simulink library "goose_lib"  (Simulink 8.1)
settings: Solver=ode45  StartTime=0.0  StopTime=10.0  RelTol=1e-3
undefined symbols (not defined in the file): CD, relay_iec61850
libraries: rtio_iec61850 x60
(part 2 of 2)

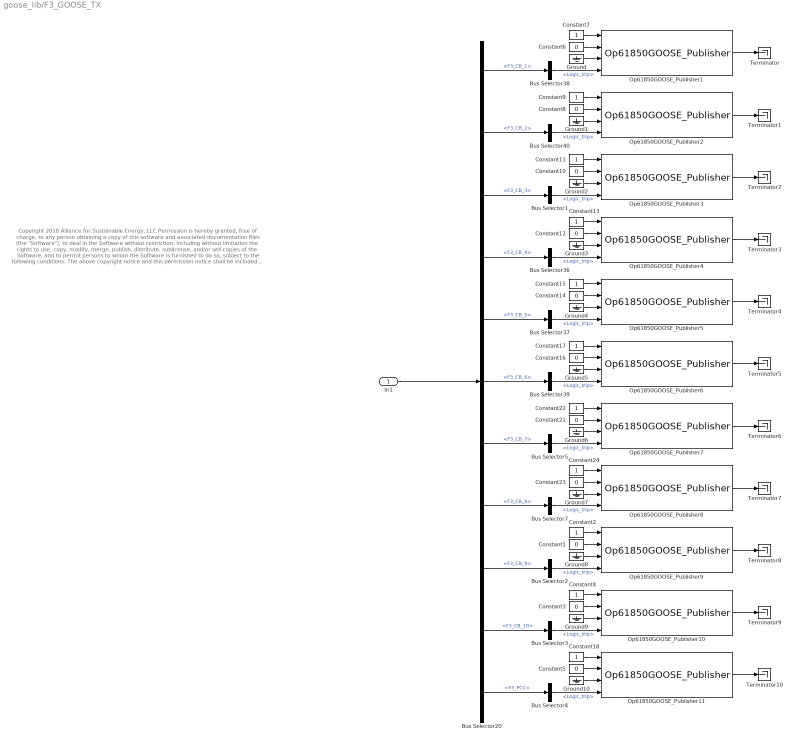
== system goose_lib/F3_GOOSE_TX ==
  note: Copyright 2018 Alliance for Sustainable Energy, LLC
      |
      | Permission is hereby granted, free of charge, to any person obtaining a copy of this software
      | and associated documentation files (the "Software"), to deal in the Software without restriction,
      | including without limitation the rights to use, copy, modify, merge, publish, distribute, sublicense,
      | and/or sell copies of the Software, and to permit persons to whom the Software is furnished to do so,
      | subject to the following conditions:
      |
      | The above copyright notice and this permission notice shall be included in all copies or substantial portions of the Software.
      |
      | THE SOFTWARE IS PROVIDED "AS IS", WITHOUT WARRANTY OF ANY KIND, EXPRESS OR IMPLIED, INCLUDING
      | BUT NOT LIMITED TO THE WARRANTIES OF MERCHANTABILITY, FITNESS FOR A PARTICULAR PURPOSE AND
      | NONINFRINGEMENT. IN NO EVENT SHALL THE AUTHORS, THE COPYRIGHT HOLDERS, THE UNITED STATES,
      | THE UNITED STATES DEPARTMENT OF ENERGY, OR ANY OF THEIR EMPLOYEES BE LIABLE FOR ANY CLAIM,
      | DAMAGES OR OTHER LIABILITY, WHETHER IN AN ACTION OF CONTRACT, TORT OR OTHERWISE, ARISING FROM,
      | OUT OF OR IN CONNECTION WITH THE SOFTWARE OR THE USE OR OTHER DEALINGS IN THE SOFTWARE.
  In1 : Inport
  Bus Selector{1..5,7,36..40} (11 alike) : BusSelector  OutputSignals=Logic_trip
  Bus Selector20 : BusSelector  OutputSignals=F3_CB_1,F3_CB_2,F3_CB_3,F3_CB_4,F3_CB_5,F3_CB_6,F3_CB_7,F3_CB_8,F3_CB_9,F3_CB_10,F3_PCC
  Constant{1,3,5..6,8,10,12,14,16,21,23} (11 alike) : Constant  Value=0
  Constant{2,4,7,9,11,13,15,17..18,22,24} (11 alike) : Constant
  Ground{,1..10} (11 alike) : Ground
  Op61850GOOSE_Publisher1 : rtio_iec61850/Op61850GOOSE_Publisher  nic_name=eth1  ied_name=CB301  select_scl=off  scl_file=CB301.icd  scl_fullpath=.\relay_iec61850  goose_name=Goose_TRIP1  goose_msgid=0x0301  mac_address=01-0C-CD-01-23-01  vlan_prio=4  vlan_id=000  mintime=25  maxtime=250  gocbref=CB301LDevice1/LLN0$GO$CB_Goose_TRIP1  dataset=CB301LDevice1/LLN0$Goose_TRIP1  goID=Goose_TRIP1  confrev=1  externalClock=off
      settings: AttributesFormatString=%<Name>\nAppId = %<goose_msgid>
  Op61850GOOSE_Publisher10 : rtio_iec61850/Op61850GOOSE_Publisher  nic_name=eth1  ied_name=CB310  select_scl=off  scl_file=CB310.icd  scl_fullpath=.\relay_iec61850  goose_name=Goose_TRIP1  goose_msgid=0x0310  mac_address=01-0C-CD-01-23-10  vlan_prio=4  vlan_id=000  mintime=25  maxtime=250  gocbref=CB310LDevice1/LLN0$GO$CB_Goose_TRIP1  dataset=CB310LDevice1/LLN0$Goose_TRIP1  goID=Goose_TRIP1  confrev=1  externalClock=off
      settings: AttributesFormatString=%<Name>\nAppId = %<goose_msgid>
  Op61850GOOSE_Publisher11 : rtio_iec61850/Op61850GOOSE_Publisher  nic_name=eth1  ied_name=CB300  select_scl=off  scl_file=CB300.icd  scl_fullpath=.\relay_iec61850  goose_name=Goose_TRIP1  goose_msgid=0x0300  mac_address=01-0C-CD-01-23-00  vlan_prio=4  vlan_id=000  mintime=25  maxtime=250  gocbref=CB300LDevice1/LLN0$GO$CB_Goose_TRIP1  dataset=CB300LDevice1/LLN0$Goose_TRIP1  goID=Goose_TRIP1  confrev=1  externalClock=off
      settings: AttributesFormatString=%<Name>\nAppId = %<goose_msgid>
  Op61850GOOSE_Publisher2 : rtio_iec61850/Op61850GOOSE_Publisher  nic_name=eth1  ied_name=CB302  select_scl=off  scl_file=CB302.icd  scl_fullpath=.\relay_iec61850  goose_name=Goose_TRIP1  goose_msgid=0x0302  mac_address=01-0C-CD-01-23-02  vlan_prio=4  vlan_id=000  mintime=25  maxtime=250  gocbref=CB302LDevice1/LLN0$GO$CB_Goose_TRIP1  dataset=CB302LDevice1/LLN0$Goose_TRIP1  goID=Goose_TRIP1  confrev=1  externalClock=off
      settings: AttributesFormatString=%<Name>\nAppId = %<goose_msgid>
  Op61850GOOSE_Publisher3 : rtio_iec61850/Op61850GOOSE_Publisher  nic_name=eth1  ied_name=CB303  select_scl=off  scl_file=CB303.icd  scl_fullpath=.\relay_iec61850  goose_name=Goose_TRIP1  goose_msgid=0x0303  mac_address=01-0C-CD-01-23-03  vlan_prio=4  vlan_id=000  mintime=25  maxtime=250  gocbref=CB303LDevice1/LLN0$GO$CB_Goose_TRIP1  dataset=CB303LDevice1/LLN0$Goose_TRIP1  goID=Goose_TRIP1  confrev=1  externalClock=off
      settings: AttributesFormatString=%<Name>\nAppId = %<goose_msgid>
  Op61850GOOSE_Publisher4 : rtio_iec61850/Op61850GOOSE_Publisher  nic_name=eth1  ied_name=CB304  select_scl=off  scl_file=CB304.icd  scl_fullpath=.\relay_iec61850  goose_name=Goose_TRIP1  goose_msgid=0x0304  mac_address=01-0C-CD-01-23-04  vlan_prio=4  vlan_id=000  mintime=25  maxtime=250  gocbref=CB304LDevice1/LLN0$GO$CB_Goose_TRIP1  dataset=CB304LDevice1/LLN0$Goose_TRIP1  goID=Goose_TRIP1  confrev=1  externalClock=off
      settings: AttributesFormatString=%<Name>\nAppId = %<goose_msgid>
  Op61850GOOSE_Publisher5 : rtio_iec61850/Op61850GOOSE_Publisher  nic_name=eth1  ied_name=CB305  select_scl=off  scl_file=CB305.icd  scl_fullpath=.\relay_iec61850  goose_name=Goose_TRIP1  goose_msgid=0x0305  mac_address=01-0C-CD-01-23-05  vlan_prio=4  vlan_id=000  mintime=25  maxtime=250  gocbref=CB305LDevice1/LLN0$GO$CB_Goose_TRIP1  dataset=CB305LDevice1/LLN0$Goose_TRIP1  goID=Goose_TRIP1  confrev=1  externalClock=off
      settings: AttributesFormatString=%<Name>\nAppId = %<goose_msgid>
  Op61850GOOSE_Publisher6 : rtio_iec61850/Op61850GOOSE_Publisher  nic_name=eth1  ied_name=CB306  select_scl=off  scl_file=CB306.icd  scl_fullpath=.\relay_iec61850  goose_name=Goose_TRIP1  goose_msgid=0x0306  mac_address=01-0C-CD-01-23-06  vlan_prio=4  vlan_id=000  mintime=25  maxtime=250  gocbref=CB306LDevice1/LLN0$GO$CB_Goose_TRIP1  dataset=CB306LDevice1/LLN0$Goose_TRIP1  goID=Goose_TRIP1  confrev=1  externalClock=off
      settings: AttributesFormatString=%<Name>\nAppId = %<goose_msgid>
  Op61850GOOSE_Publisher7 : rtio_iec61850/Op61850GOOSE_Publisher  nic_name=eth1  ied_name=CB307  select_scl=off  scl_file=CB307.icd  scl_fullpath=.\relay_iec61850  goose_name=Goose_TRIP1  goose_msgid=0x0307  mac_address=01-0C-CD-01-23-07  vlan_prio=4  vlan_id=000  mintime=25  maxtime=250  gocbref=CB307LDevice1/LLN0$GO$CB_Goose_TRIP1  dataset=CB307LDevice1/LLN0$Goose_TRIP1  goID=Goose_TRIP1  confrev=1  externalClock=off
      settings: AttributesFormatString=%<Name>\nAppId = %<goose_msgid>
  Op61850GOOSE_Publisher8 : rtio_iec61850/Op61850GOOSE_Publisher  nic_name=eth1  ied_name=CB308  select_scl=off  scl_file=CB308.icd  scl_fullpath=.\relay_iec61850  goose_name=Goose_TRIP1  goose_msgid=0x0308  mac_address=01-0C-CD-01-23-08  vlan_prio=4  vlan_id=000  mintime=25  maxtime=250  gocbref=CB308LDevice1/LLN0$GO$CB_Goose_TRIP1  dataset=CB308LDevice1/LLN0$Goose_TRIP1  goID=Goose_TRIP1  confrev=1  externalClock=off
      settings: AttributesFormatString=%<Name>\nAppId = %<goose_msgid>
  Op61850GOOSE_Publisher9 : rtio_iec61850/Op61850GOOSE_Publisher  nic_name=eth1  ied_name=CB309  select_scl=off  scl_file=CB309.icd  scl_fullpath=.\relay_iec61850  goose_name=Goose_TRIP1  goose_msgid=0x0309  mac_address=01-0C-CD-01-23-09  vlan_prio=4  vlan_id=000  mintime=25  maxtime=250  gocbref=CB309LDevice1/LLN0$GO$CB_Goose_TRIP1  dataset=CB309LDevice1/LLN0$Goose_TRIP1  goID=Goose_TRIP1  confrev=1  externalClock=off
      settings: AttributesFormatString=%<Name>\nAppId = %<goose_msgid>
  Terminator{,1..10} (11 alike) : Terminator
  wires:
  Ground5/1 -> Op61850GOOSE_Publisher6/3
  Constant17/1 -> Op61850GOOSE_Publisher6/1
  Ground3/1 -> Op61850GOOSE_Publisher4/3
  Ground1/1 -> Op61850GOOSE_Publisher2/3
  In1/1 -> Bus Selector20/1
  Constant16/1 -> Op61850GOOSE_Publisher6/2
  Bus Selector39/1 -> Op61850GOOSE_Publisher6/4  "<Logic_trip>"
  Bus Selector20/6 -> Bus Selector39/1  "<F3_CB_6>"
  Op61850GOOSE_Publisher5/1 -> Terminator4/1
  Ground4/1 -> Op61850GOOSE_Publisher5/3
  Constant12/1 -> Op61850GOOSE_Publisher4/2
  Constant13/1 -> Op61850GOOSE_Publisher4/1
  Bus Selector36/1 -> Op61850GOOSE_Publisher4/4  "<Logic_trip>"
  Bus Selector20/4 -> Bus Selector36/1  "<F3_CB_4>"
  Op61850GOOSE_Publisher3/1 -> Terminator2/1
  Constant9/1 -> Op61850GOOSE_Publisher2/1
  Constant8/1 -> Op61850GOOSE_Publisher2/2
  Bus Selector40/1 -> Op61850GOOSE_Publisher2/4  "<Logic_trip>"
  Bus Selector20/2 -> Bus Selector40/1  "<F3_CB_2>"
  Ground2/1 -> Op61850GOOSE_Publisher3/3
  Op61850GOOSE_Publisher1/1 -> Terminator/1
  Op61850GOOSE_Publisher2/1 -> Terminator1/1
  Op61850GOOSE_Publisher4/1 -> Terminator3/1
  Constant14/1 -> Op61850GOOSE_Publisher5/2
  Constant7/1 -> Op61850GOOSE_Publisher1/1
  Ground/1 -> Op61850GOOSE_Publisher1/3
  Constant11/1 -> Op61850GOOSE_Publisher3/1
  Constant10/1 -> Op61850GOOSE_Publisher3/2
  Constant15/1 -> Op61850GOOSE_Publisher5/1
  Bus Selector37/1 -> Op61850GOOSE_Publisher5/4  "<Logic_trip>"
  Bus Selector20/5 -> Bus Selector37/1  "<F3_CB_5>"
  Bus Selector38/1 -> Op61850GOOSE_Publisher1/4  "<Logic_trip>"
  Bus Selector20/1 -> Bus Selector38/1  "<F3_CB_1>"
  Bus Selector20/3 -> Bus Selector1/1  "<F3_CB_3>"
  Bus Selector1/1 -> Op61850GOOSE_Publisher3/4  "<Logic_trip>"
  Constant6/1 -> Op61850GOOSE_Publisher1/2
  Op61850GOOSE_Publisher6/1 -> Terminator5/1
  Ground9/1 -> Op61850GOOSE_Publisher10/3
  Ground7/1 -> Op61850GOOSE_Publisher8/3
  Op61850GOOSE_Publisher11/1 -> Terminator10/1
  Ground10/1 -> Op61850GOOSE_Publisher11/3
  Constant3/1 -> Op61850GOOSE_Publisher10/2
  Constant4/1 -> Op61850GOOSE_Publisher10/1
  Bus Selector3/1 -> Op61850GOOSE_Publisher10/4  "<Logic_trip>"
  Op61850GOOSE_Publisher9/1 -> Terminator8/1
  Constant24/1 -> Op61850GOOSE_Publisher8/1
  Constant23/1 -> Op61850GOOSE_Publisher8/2
  Bus Selector7/1 -> Op61850GOOSE_Publisher8/4  "<Logic_trip>"
  Ground8/1 -> Op61850GOOSE_Publisher9/3
  Op61850GOOSE_Publisher7/1 -> Terminator6/1
  Op61850GOOSE_Publisher8/1 -> Terminator7/1
  Op61850GOOSE_Publisher10/1 -> Terminator9/1
  Constant5/1 -> Op61850GOOSE_Publisher11/2
  Constant22/1 -> Op61850GOOSE_Publisher7/1
  Ground6/1 -> Op61850GOOSE_Publisher7/3
  Constant2/1 -> Op61850GOOSE_Publisher9/1
  Constant1/1 -> Op61850GOOSE_Publisher9/2
  Constant18/1 -> Op61850GOOSE_Publisher11/1
  Bus Selector4/1 -> Op61850GOOSE_Publisher11/4  "<Logic_trip>"
  Bus Selector5/1 -> Op61850GOOSE_Publisher7/4  "<Logic_trip>"
  Bus Selector2/1 -> Op61850GOOSE_Publisher9/4  "<Logic_trip>"
  Constant21/1 -> Op61850GOOSE_Publisher7/2
  Bus Selector20/10 -> Bus Selector3/1  "<F3_CB_10>"
  Bus Selector20/8 -> Bus Selector7/1  "<F3_CB_8>"
  Bus Selector20/11 -> Bus Selector4/1  "<F3_PCC>"
  Bus Selector20/7 -> Bus Selector5/1  "<F3_CB_7>"
  Bus Selector20/9 -> Bus Selector2/1  "<F3_CB_9>"

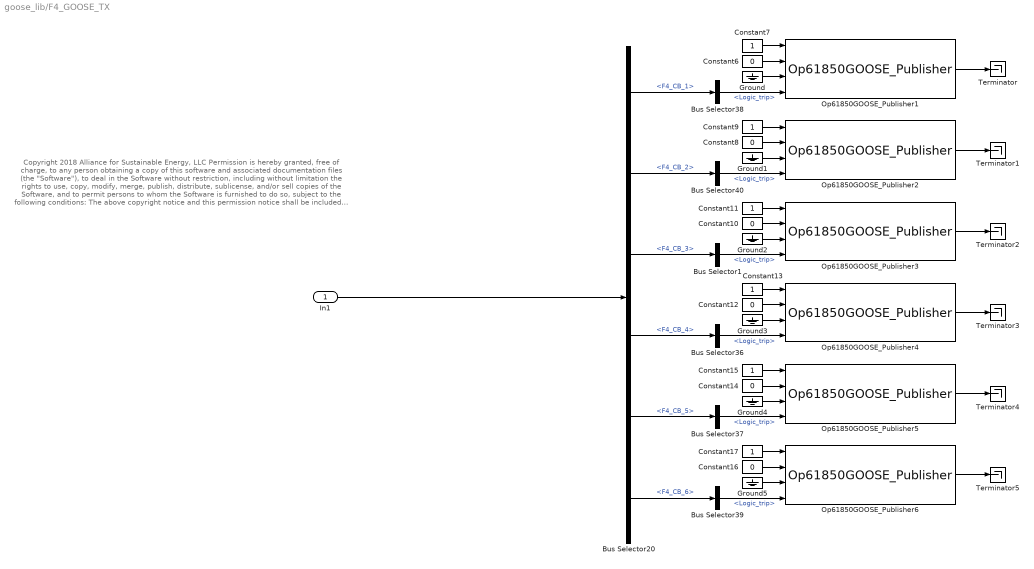
== system goose_lib/F4_GOOSE_TX ==
  note: Copyright 2018 Alliance for Sustainable Energy, LLC
      |
      | Permission is hereby granted, free of charge, to any person obtaining a copy of this software
      | and associated documentation files (the "Software"), to deal in the Software without restriction,
      | including without limitation the rights to use, copy, modify, merge, publish, distribute, sublicense,
      | and/or sell copies of the Software, and to permit persons to whom the Software is furnished to do so,
      | subject to the following conditions:
      |
      | The above copyright notice and this permission notice shall be included in all copies or substantial portions of the Software.
      |
      | THE SOFTWARE IS PROVIDED "AS IS", WITHOUT WARRANTY OF ANY KIND, EXPRESS OR IMPLIED, INCLUDING
      | BUT NOT LIMITED TO THE WARRANTIES OF MERCHANTABILITY, FITNESS FOR A PARTICULAR PURPOSE AND
      | NONINFRINGEMENT. IN NO EVENT SHALL THE AUTHORS, THE COPYRIGHT HOLDERS, THE UNITED STATES,
      | THE UNITED STATES DEPARTMENT OF ENERGY, OR ANY OF THEIR EMPLOYEES BE LIABLE FOR ANY CLAIM,
      | DAMAGES OR OTHER LIABILITY, WHETHER IN AN ACTION OF CONTRACT, TORT OR OTHERWISE, ARISING FROM,
      | OUT OF OR IN CONNECTION WITH THE SOFTWARE OR THE USE OR OTHER DEALINGS IN THE SOFTWARE.
  In1 : Inport
  Bus Selector{1,36..40} (6 alike) : BusSelector  OutputSignals=Logic_trip
  Bus Selector20 : BusSelector  OutputSignals=F4_CB_1,F4_CB_2,F4_CB_3,F4_CB_4,F4_CB_5,F4_CB_6
  Constant{6,8,10,12,14,16} (6 alike) : Constant  Value=0
  Constant{7,9,11,13,15,17} (6 alike) : Constant
  Ground{,1..5} (6 alike) : Ground
  Op61850GOOSE_Publisher1 : rtio_iec61850/Op61850GOOSE_Publisher  nic_name=eth1  ied_name=CB401  select_scl=off  scl_file=CB401.icd  scl_fullpath=.\relay_iec61850  goose_name=Goose_TRIP1  goose_msgid=0x0401  mac_address=01-0C-CD-01-24-01  vlan_prio=4  vlan_id=000  mintime=25  maxtime=250  gocbref=CB401LDevice1/LLN0$GO$CB_Goose_TRIP1  dataset=CB401LDevice1/LLN0$Goose_TRIP1  goID=Goose_TRIP1  confrev=1  externalClock=off
      settings: AttributesFormatString=%<Name>\nAppId = %<goose_msgid>
  Op61850GOOSE_Publisher2 : rtio_iec61850/Op61850GOOSE_Publisher  nic_name=eth1  ied_name=CB402  select_scl=off  scl_file=CB402.icd  scl_fullpath=.\relay_iec61850  goose_name=Goose_TRIP1  goose_msgid=0x0402  mac_address=01-0C-CD-01-24-02  vlan_prio=4  vlan_id=000  mintime=25  maxtime=250  gocbref=CB402LDevice1/LLN0$GO$CB_Goose_TRIP1  dataset=CB402LDevice1/LLN0$Goose_TRIP1  goID=Goose_TRIP1  confrev=1  externalClock=off
      settings: AttributesFormatString=%<Name>\nAppId = %<goose_msgid>
  Op61850GOOSE_Publisher3 : rtio_iec61850/Op61850GOOSE_Publisher  nic_name=eth1  ied_name=CB403  select_scl=off  scl_file=CB403.icd  scl_fullpath=.\relay_iec61850  goose_name=Goose_TRIP1  goose_msgid=0x0403  mac_address=01-0C-CD-01-24-03  vlan_prio=4  vlan_id=000  mintime=25  maxtime=250  gocbref=CB403LDevice1/LLN0$GO$CB_Goose_TRIP1  dataset=CB403LDevice1/LLN0$Goose_TRIP1  goID=Goose_TRIP1  confrev=1  externalClock=off
      settings: AttributesFormatString=%<Name>\nAppId = %<goose_msgid>
  Op61850GOOSE_Publisher4 : rtio_iec61850/Op61850GOOSE_Publisher  nic_name=eth1  ied_name=CB404  select_scl=off  scl_file=CB404.icd  scl_fullpath=.\relay_iec61850  goose_name=Goose_TRIP1  goose_msgid=0x0404  mac_address=01-0C-CD-01-24-04  vlan_prio=4  vlan_id=000  mintime=25  maxtime=250  gocbref=CB404LDevice1/LLN0$GO$CB_Goose_TRIP1  dataset=CB404LDevice1/LLN0$Goose_TRIP1  goID=Goose_TRIP1  confrev=1  externalClock=off
      settings: AttributesFormatString=%<Name>\nAppId = %<goose_msgid>
  Op61850GOOSE_Publisher5 : rtio_iec61850/Op61850GOOSE_Publisher  nic_name=eth1  ied_name=CB405  select_scl=off  scl_file=CB405.icd  scl_fullpath=.\relay_iec61850  goose_name=Goose_TRIP1  goose_msgid=0x0405  mac_address=01-0C-CD-01-24-05  vlan_prio=4  vlan_id=000  mintime=25  maxtime=250  gocbref=CB405LDevice1/LLN0$GO$CB_Goose_TRIP1  dataset=CB405LDevice1/LLN0$Goose_TRIP1  goID=Goose_TRIP1  confrev=1  externalClock=off
      settings: AttributesFormatString=%<Name>\nAppId = %<goose_msgid>
  Op61850GOOSE_Publisher6 : rtio_iec61850/Op61850GOOSE_Publisher  nic_name=eth1  ied_name=CB406  select_scl=off  scl_file=CB406.icd  scl_fullpath=.\relay_iec61850  goose_name=Goose_TRIP1  goose_msgid=0x0406  mac_address=01-0C-CD-01-24-06  vlan_prio=4  vlan_id=000  mintime=25  maxtime=250  gocbref=CB406LDevice1/LLN0$GO$CB_Goose_TRIP1  dataset=CB406LDevice1/LLN0$Goose_TRIP1  goID=Goose_TRIP1  confrev=1  externalClock=off
      settings: AttributesFormatString=%<Name>\nAppId = %<goose_msgid>
  Terminator{,1..5} (6 alike) : Terminator
  wires:
  Op61850GOOSE_Publisher6/1 -> Terminator5/1
  Constant6/1 -> Op61850GOOSE_Publisher1/2
  Bus Selector1/1 -> Op61850GOOSE_Publisher3/4  "<Logic_trip>"
  Bus Selector20/3 -> Bus Selector1/1  "<F4_CB_3>"
  Bus Selector20/1 -> Bus Selector38/1  "<F4_CB_1>"
  Bus Selector38/1 -> Op61850GOOSE_Publisher1/4  "<Logic_trip>"
  Bus Selector20/5 -> Bus Selector37/1  "<F4_CB_5>"
  Bus Selector37/1 -> Op61850GOOSE_Publisher5/4  "<Logic_trip>"
  Constant15/1 -> Op61850GOOSE_Publisher5/1
  Constant10/1 -> Op61850GOOSE_Publisher3/2
  Constant11/1 -> Op61850GOOSE_Publisher3/1
  Ground/1 -> Op61850GOOSE_Publisher1/3
  Constant7/1 -> Op61850GOOSE_Publisher1/1
  Constant14/1 -> Op61850GOOSE_Publisher5/2
  Op61850GOOSE_Publisher4/1 -> Terminator3/1
  Op61850GOOSE_Publisher2/1 -> Terminator1/1
  Op61850GOOSE_Publisher1/1 -> Terminator/1
  Ground2/1 -> Op61850GOOSE_Publisher3/3
  Bus Selector20/2 -> Bus Selector40/1  "<F4_CB_2>"
  Bus Selector40/1 -> Op61850GOOSE_Publisher2/4  "<Logic_trip>"
  Constant8/1 -> Op61850GOOSE_Publisher2/2
  Constant9/1 -> Op61850GOOSE_Publisher2/1
  Op61850GOOSE_Publisher3/1 -> Terminator2/1
  Bus Selector20/4 -> Bus Selector36/1  "<F4_CB_4>"
  Bus Selector36/1 -> Op61850GOOSE_Publisher4/4  "<Logic_trip>"
  Constant13/1 -> Op61850GOOSE_Publisher4/1
  Constant12/1 -> Op61850GOOSE_Publisher4/2
  Ground4/1 -> Op61850GOOSE_Publisher5/3
  Op61850GOOSE_Publisher5/1 -> Terminator4/1
  Bus Selector20/6 -> Bus Selector39/1  "<F4_CB_6>"
  Bus Selector39/1 -> Op61850GOOSE_Publisher6/4  "<Logic_trip>"
  Constant16/1 -> Op61850GOOSE_Publisher6/2
  In1/1 -> Bus Selector20/1
  Ground1/1 -> Op61850GOOSE_Publisher2/3
  Ground3/1 -> Op61850GOOSE_Publisher4/3
  Constant17/1 -> Op61850GOOSE_Publisher6/1
  Ground5/1 -> Op61850GOOSE_Publisher6/3

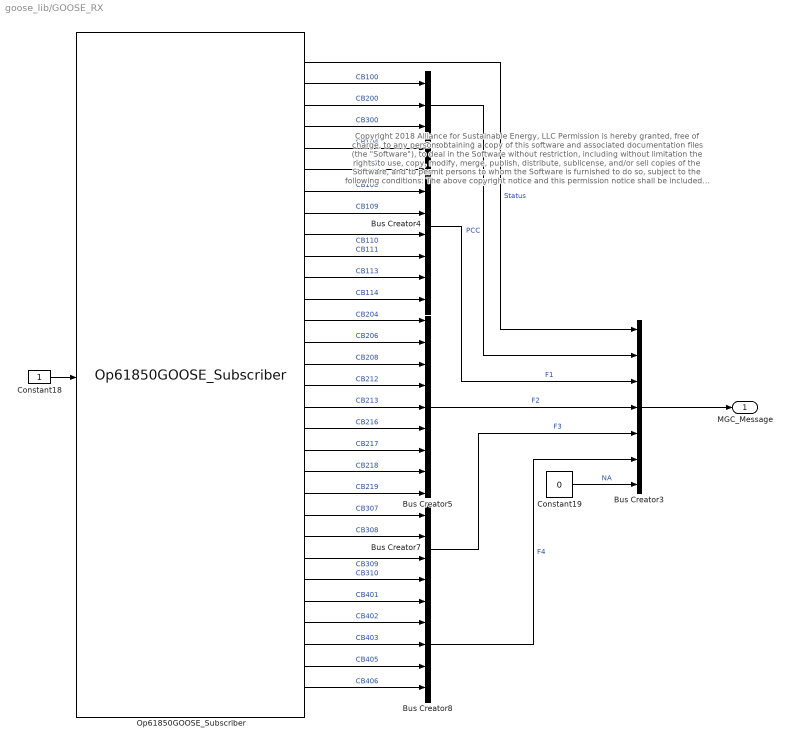
== system goose_lib/GOOSE_RX  ==
  note: Copyright 2018 Alliance for Sustainable Energy, LLC
      |
      | Permission is hereby granted, free of charge, to any person obtaining a copy of this software
      | and associated documentation files (the "Software"), to deal in the Software without restriction,
      | including without limitation the rights to use, copy, modify, merge, publish, distribute, sublicense,
      | and/or sell copies of the Software, and to permit persons to whom the Software is furnished to do so,
      | subject to the following conditions:
      |
      | The above copyright notice and this permission notice shall be included in all copies or substantial portions of the Software.
      |
      | THE SOFTWARE IS PROVIDED "AS IS", WITHOUT WARRANTY OF ANY KIND, EXPRESS OR IMPLIED, INCLUDING
      | BUT NOT LIMITED TO THE WARRANTIES OF MERCHANTABILITY, FITNESS FOR A PARTICULAR PURPOSE AND
      | NONINFRINGEMENT. IN NO EVENT SHALL THE AUTHORS, THE COPYRIGHT HOLDERS, THE UNITED STATES,
      | THE UNITED STATES DEPARTMENT OF ENERGY, OR ANY OF THEIR EMPLOYEES BE LIABLE FOR ANY CLAIM,
      | DAMAGES OR OTHER LIABILITY, WHETHER IN AN ACTION OF CONTRACT, TORT OR OTHERWISE, ARISING FROM,
      | OUT OF OR IN CONNECTION WITH THE SOFTWARE OR THE USE OR OTHER DEALINGS IN THE SOFTWARE.
  Bus Creator2 : BusCreator  Inputs=3
  Bus Creator3 : BusCreator  Inputs=7
  Bus Creator4 : BusCreator  Inputs=8
  Bus Creator5 : BusCreator  Inputs=9
  Bus Creator7 : BusCreator
  Bus Creator8 : BusCreator  Inputs=5
  Constant18 : Constant
  Constant19 : Constant  Value=0
  Op61850GOOSE_Subscriber : rtio_iec61850/Op61850GOOSE_Subscriber  nic_name=eth1  ied_name=MGC  select_scl=off  scl_file=MGC.ICD  scl_fullpath=.\relay_iec61850  goose_name=Goose_MGCcmd  goose_msgid=0x0001  mac_address=01-0C-CD-01-28-60
      settings: AttributesFormatString=%<Name>\nAppId = %<goose_msgid>
  MGC_Message : Outport
  wires:
  Op61850GOOSE_Subscriber/26 -> Bus Creator8/1  "CB401"
  Op61850GOOSE_Subscriber/27 -> Bus Creator8/2  "CB402"
  Op61850GOOSE_Subscriber/29 -> Bus Creator8/4  "CB405"
  Constant19/1 -> Bus Creator3/7  "NA"
  Op61850GOOSE_Subscriber/22 -> Bus Creator7/1  "CB307"
  Op61850GOOSE_Subscriber/23 -> Bus Creator7/2  "CB308"
  Op61850GOOSE_Subscriber/24 -> Bus Creator7/3  "CB309"
  Op61850GOOSE_Subscriber/25 -> Bus Creator7/4  "CB310"
  Bus Creator7/1 -> Bus Creator3/5  "F3"
  Op61850GOOSE_Subscriber/28 -> Bus Creator8/3  "CB403"
  Op61850GOOSE_Subscriber/30 -> Bus Creator8/5  "CB406"
  Bus Creator8/1 -> Bus Creator3/6  "F4"
  Bus Creator5/1 -> Bus Creator3/4  "F2"
  Op61850GOOSE_Subscriber/14 -> Bus Creator5/2  "CB206"
  Op61850GOOSE_Subscriber/16 -> Bus Creator5/4  "CB212"
  Op61850GOOSE_Subscriber/13 -> Bus Creator5/1  "CB204"
  Op61850GOOSE_Subscriber/15 -> Bus Creator5/3  "CB208"
  Op61850GOOSE_Subscriber/20 -> Bus Creator5/8  "CB218"
  Op61850GOOSE_Subscriber/17 -> Bus Creator5/5  "CB213"
  Op61850GOOSE_Subscriber/19 -> Bus Creator5/7  "CB217"
  Op61850GOOSE_Subscriber/18 -> Bus Creator5/6  "CB216"
  Op61850GOOSE_Subscriber/21 -> Bus Creator5/9  "CB219"
  Bus Creator4/1 -> Bus Creator3/3  "F1"
  Op61850GOOSE_Subscriber/12 -> Bus Creator4/8  "CB114"
  Op61850GOOSE_Subscriber/11 -> Bus Creator4/7  "CB113"
  Op61850GOOSE_Subscriber/10 -> Bus Creator4/6  "CB111"
  Op61850GOOSE_Subscriber/5 -> Bus Creator4/1  "CB104"
  Op61850GOOSE_Subscriber/9 -> Bus Creator4/5  "CB110"
  Op61850GOOSE_Subscriber/6 -> Bus Creator4/2  "CB107"
  Op61850GOOSE_Subscriber/8 -> Bus Creator4/4  "CB109"
  Op61850GOOSE_Subscriber/7 -> Bus Creator4/3  "CB108"
  Bus Creator2/1 -> Bus Creator3/2  "PCC"
  Op61850GOOSE_Subscriber/4 -> Bus Creator2/3  "CB300"
  Op61850GOOSE_Subscriber/3 -> Bus Creator2/2  "CB200"
  Op61850GOOSE_Subscriber/2 -> Bus Creator2/1  "CB100"
  Bus Creator3/1 -> MGC_Message/1
  Op61850GOOSE_Subscriber/1 -> Bus Creator3/1  "Status"
  Constant18/1 -> Op61850GOOSE_Subscriber/1
